simulink model "General_posicion1"  (R2020b)
settings: Solver=ode5  StartTime=0.0  StopTime=inf  RelTol=1e-3
undefined symbols (not defined in the file): National_Instruments, PCI
libraries: simulink x4, pid_lib x3, fuzblock x2, sldrtlib x2
settings Model: SimulationMode=external  Creator=Usuario_UMA  LastModifiedBy=alumnoic06
settings RTWCC: Description=Simulink Desktop Real-Time  SystemTargetFile=sldrt.tlc  TemplateMakefile=sldrt.tmf  RTWCompilerOptimization=on
settings CodeAppCC: MaxIdLength=95
settings SimulinkDesktopRealTimeCC: TargetPreCompLibLocation=C:\Program Files\MATLAB\R2020\toolbox\sldrt\lib\win64

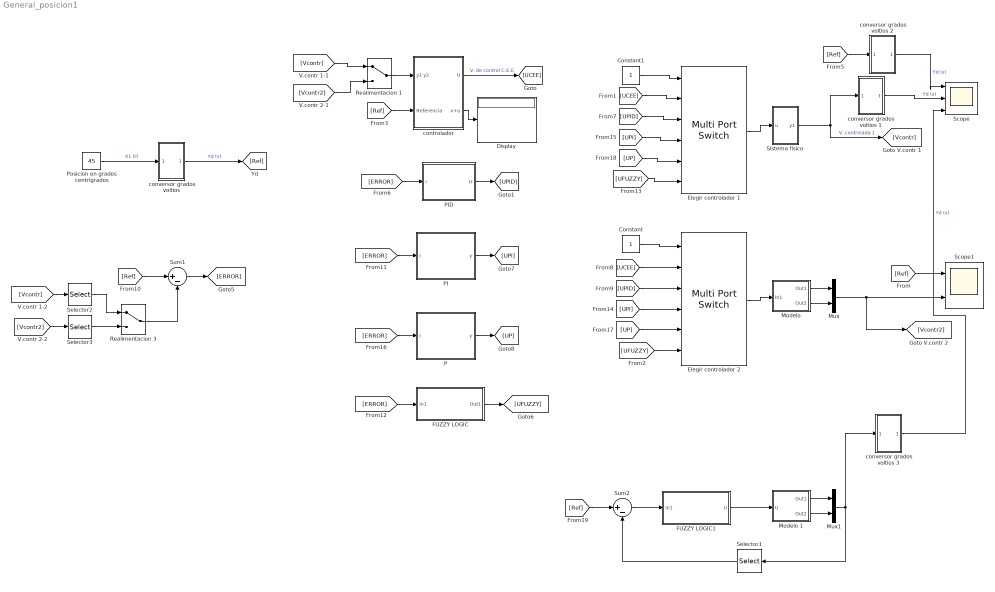
== system General_posicion1 ==
  Constant : Constant
  Constant1 : Constant
  Display : Display
  Elegir controlador 1 : MultiPortSwitch  Inputs=5
  Elegir controlador 2 : MultiPortSwitch  Inputs=5
  FUZZY LOGIC : Subsystem
  FUZZY LOGIC1 : Subsystem
  "Modelo " : Subsystem
  Modelo 1 : Subsystem
  Mux : Mux  Inputs=2
  Mux1 : Mux  Inputs=2
  P : Subsystem
  PI : Subsystem
  PID : Subsystem
  Posicion en grados centrigrados : Constant  Value=45
  Realimentacion 1 : ManualSwitch
  Realimentacion 3 : ManualSwitch
  Scope : Scope  NumInputPorts=3
  Scope1 : Scope  NumInputPorts=2
  Selector1 : Selector  InputPortWidth=2  IndexOptions=Index vector (dialog)  Indices=[1]  OutputSizes=1
  Selector2 : Selector  InputPortWidth=2  IndexOptions=Index vector (dialog)  Indices=[1]  OutputSizes=1
  Selector3 : Selector  InputPortWidth=2  IndexOptions=Index vector (dialog)  Indices=[1]  OutputSizes=1
  Sistema fisico : Subsystem
  Sum1 : Sum  Inputs=|+-
  Sum2 : Sum  Inputs=|+-
  controlador : Subsystem
  "conversor grados voltios " : Subsystem  mask{a=4.91, b=0}
  conversor grados voltios 1 : Subsystem  mask{a=4.91, b=0}
  conversor grados voltios 2 : Subsystem  mask{a=4.91, b=0}
  conversor grados voltios 3 : Subsystem  mask{a=4.91, b=0}
  wires:
  Posicion en grados centrigrados/1 -> "conversor grados voltios "/1(In1)  "X1 (º)"
  controlador/2(x+u) -> Display/1
  Sistema fisico/1(y1) -> conversor grados voltios 1/1(In1), [Vcontr]  "V. controlada 1"
  "conversor grados voltios "/1(Out1) -> [Ref]  "Yd (v)"
  controlador/1(U) -> [UCEE]  "V. de control C:E:E"
  "Modelo "/1(Out1) -> Mux/1
  "Modelo "/2(Out2) -> Mux/2
  Mux/1 -> [Vcontr2], Scope1/2
  Realimentacion 1/1 -> controlador/1(y1 y2)
  [Ref] -> Scope1/1
  [Vcontr] -> Realimentacion 1/1
  [Vcontr2] -> Realimentacion 1/2
  [Ref] -> controlador/2(Referencia)
  Elegir controlador 2/1 -> "Modelo "/1(In1)
  Elegir controlador 1/1 -> Sistema fisico/1(u)
  PID/1(U) -> [UPID]
  [UCEE] -> Elegir controlador 1/2
  [UPID] -> Elegir controlador 1/3
  [UCEE] -> Elegir controlador 2/2
  [UPID] -> Elegir controlador 2/3
  Constant/1 -> Elegir controlador 2/1
  Constant1/1 -> Elegir controlador 1/1
  [Vcontr2] -> Selector3/1
  Selector3/1 -> Realimentacion 3/2
  [Ref] -> Sum1/1
  Realimentacion 3/1 -> Sum1/2
  Selector2/1 -> Realimentacion 3/1
  Sum1/1 -> [ERROR]
  [Vcontr] -> Selector2/1
  [ERROR] -> PID/1(r)
  [ERROR] -> FUZZY LOGIC/1(In1)
  FUZZY LOGIC/1(Out1) -> [UFUZZY]
  [UFUZZY] -> Elegir controlador 2/6
  [UFUZZY] -> Elegir controlador 1/6
  [ERROR] -> PI/1(r)
  PI/1(y) -> [UPI]
  [UPI] -> Elegir controlador 2/4
  [UPI] -> Elegir controlador 1/4
  [ERROR] -> P/1(r)
  P/1(y) -> [UP]
  [UP] -> Elegir controlador 2/5
  [UP] -> Elegir controlador 1/5
  conversor grados voltios 1/1(Out1) -> Scope/2  "Yd (v)"
  [Ref] -> conversor grados voltios 2/1(In1)
  conversor grados voltios 2/1(Out1) -> Scope/1  "Yd (v)"
  [Ref] -> Sum2/1
  Modelo 1/2(Out2) -> Mux1/2
  Modelo 1/1(Out1) -> Mux1/1
  Selector1/1 -> Sum2/2
  Mux1/1 -> Selector1/1, conversor grados voltios 3/1(In1)
  conversor grados voltios 3/1(Out1) -> Scope/3  "Yd (v)"
  Sum2/1 -> FUZZY LOGIC1/1(In1)
  FUZZY LOGIC1/1(U) -> Modelo 1/1(U)

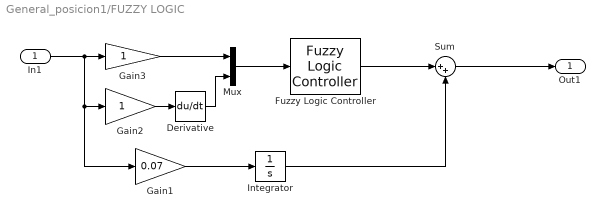
== system General_posicion1/FUZZY LOGIC ==
  In1 : Inport
  Derivative : Derivative
  Fuzzy Logic Controller : fuzblock/Fuzzy Logic  Controller  FIS='FUZZY1b.fis'  OutputSampleNumber=101  DataType=double  FuzzifiedInputs=off  RuleFiringStrengths=off  RuleOutputs=off  AggregatedOutputs=off  SimulateUsing=Interpreted execution  OutOfRangeInputValueMessage=warning  NoRuleFiredMessage=warning  EmptyOutputFuzzySetMessage=warning
  Gain1 : Gain  Gain=0.07
  Gain2 : Gain
  Gain3 : Gain
  Integrator : Integrator
  Mux : Mux  Inputs=2
  Sum : Sum  Inputs=|++
  Out1 : Outport
  wires:
  Derivative/1 -> Mux/2
  In1/1 -> Gain3/1, Gain1/1, Gain2/1
  Mux/1 -> Fuzzy Logic Controller/1
  Gain3/1 -> Mux/1
  Gain2/1 -> Derivative/1
  Gain1/1 -> Integrator/1
  Fuzzy Logic Controller/1 -> Sum/1
  Sum/1 -> Out1/1
  Integrator/1 -> Sum/2

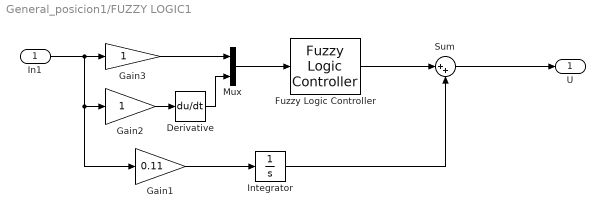
== system General_posicion1/FUZZY LOGIC1 ==
  In1 : Inport
  Derivative : Derivative
  Fuzzy Logic Controller : fuzblock/Fuzzy Logic  Controller  FIS='FUZZY1b.fis'  OutputSampleNumber=101  DataType=double  FuzzifiedInputs=off  RuleFiringStrengths=off  RuleOutputs=off  AggregatedOutputs=off  SimulateUsing=Interpreted execution  OutOfRangeInputValueMessage=warning  NoRuleFiredMessage=warning  EmptyOutputFuzzySetMessage=warning
  Gain1 : Gain  Gain=0.11
  Gain2 : Gain
  Gain3 : Gain
  Integrator : Integrator
  Mux : Mux  Inputs=2
  Sum : Sum  Inputs=|++
  U : Outport
  wires:
  Derivative/1 -> Mux/2
  In1/1 -> Gain3/1, Gain1/1, Gain2/1
  Mux/1 -> Fuzzy Logic Controller/1
  Gain3/1 -> Mux/1
  Gain2/1 -> Derivative/1
  Gain1/1 -> Integrator/1
  Fuzzy Logic Controller/1 -> Sum/1
  Sum/1 -> U/1
  Integrator/1 -> Sum/2

== system General_posicion1/Modelo  ==
  In1 : Inport
  Transfer Fcn : TransferFcn  Numerator=[114.486]  Denominator=[1 7.35 0]
  Transfer Fcn1 : TransferFcn  Numerator=[19.12]  Denominator=[1 7.35]
  Out1 : Outport
  Out2 : Outport  Port=2
  wires:
  In1/1 -> Transfer Fcn1/1, Transfer Fcn/1
  Transfer Fcn/1 -> Out1/1
  Transfer Fcn1/1 -> Out2/1

== system General_posicion1/Modelo 1 ==
  U : Inport
  Transfer Fcn : TransferFcn  Numerator=[114.486]  Denominator=[1 7.35 0]
  Transfer Fcn1 : TransferFcn  Numerator=[19.12]  Denominator=[1 7.35]
  Out1 : Outport
  Out2 : Outport  Port=2
  wires:
  U/1 -> Transfer Fcn1/1, Transfer Fcn/1
  Transfer Fcn/1 -> Out1/1
  Transfer Fcn1/1 -> Out2/1

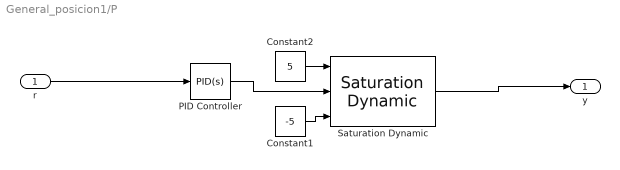
== system General_posicion1/P ==
  r : Inport
  Constant1 : Constant  Value=-5
  Constant2 : Constant  Value=5
  PID Controller : pid_lib/PID Controller  Controller=PID  Form=Parallel  TimeDomain=Continuous-time  UseExternalTs=off  SampleTime=-1  IntegratorMethod=Forward Euler  FilterMethod=Forward Euler  ControllerParametersSource=internal  P=0.5  I=0.2  D=0  UseFilter=on  N=100  TunerSelectOption=Transfer Function Based (PID Tuner App)  InitialConditionSource=internal  InitialConditionForIntegrator=0  InitialConditionForFilter=0  DifferentiatorICPrevScaledInput=0  ExternalReset=none  TrackingMode=off  Kt=1  LimitOutput=off  SatLimitsSource=internal  UpperSaturationLimit=inf  LowerSaturationLimit=-inf  LinearizeAsGain=on  AntiWindupMode=none  Kb=1  POutMin=[]  POutMax=[]  IOutMin=[]  IOutMax=[]  DOutMin=[]  DOutMax=[]  NOutMin=[]  NOutMax=[]  SumOutMin=[]  SumOutMax=[]  SaturationOutMin=[]  SaturationOutMax=[]  PParamMin=[]  PParamMax=[]  IParamMin=[]  IParamMax=[]  DParamMin=[]  DParamMax=[]  NParamMin=[]  NParamMax=[]  KbParamMin=[]  KbParamMax=[]  KtParamMin=[]  KtParamMax=[]  KbOutMin=[]  KbOutMax=[]  KtOutMin=[]  KtOutMax=[]  IntegratorOutMin=[]  IntegratorOutMax=[]  FilterOutMin=[]  FilterOutMax=[]  SumI1OutMin=[]  SumI1OutMax=[]  SumI2OutMin=[]  SumI2OutMax=[]  SumI3OutMin=[]  SumI3OutMax=[]  SumI4OutMin=[]  SumI4OutMax=[]  SumDOutMin=[]  SumDOutMax=[]  DifferentiatorOutMin=[]  DifferentiatorOutMax=[]  FilterDiffOutCoefMin=[]  FilterDiffOutCoefMax=[]  ReciprocalOutMin=[]  ReciprocalOutMax=[]  SumDenOutMin=[]  SumDenOutMax=[]  SumNumOutMin=[]  SumNumOutMax=[]  DivideOutMin=[]  DivideOutMax=[]  UdiffTsProdOutMin=[]  UdiffTsProdOutMax=[]  NTsProdOutMin=[]  NTsProdOutMax=[]  UintegralTsProdOutMin=[]  UintegralTsProdOutMax=[]  UngainTsProdOutMin=[]  UngainTsProdOutMax=[]  IntegratorContinuousStateAttributes=''  IntegratorStateMustResolveToSignalObject=off  IntegratorRTWStateStorageClass=Auto  FilterContinuousStateAttributes=''  FilterStateMustResolveToSignalObject=off  FilterRTWStateStorageClass=Auto  ParallelPVariant=InternalParameters  IdealPVariant=Disabled  IVariant=InternalParameters  DVariant=InternalParameters  IntegratorVariant=Continuous  SatVariant=Disabled  AWVariant=Passthrough  PCopyVariant=Disabled  TRVariant=Disabled  FdbkBlocksVariant=Forward  IdealPFdbkVariant=Disabled  SatFdbkVariant=Disabled  DerivativeFilterVariant=ContFilter  NVariant=InternalParameters  NCopyVariant=Disabled  FilterICVariant=InternalICsFilter  IntegratorICVariant=InternalICs  ExternalResetVariant=Disabled  TRSumVariant=Passthrough  SumFdbkVariant=Disabled  SumVariant=Sum_PID  TsampFilterVariant=InternalTs  TsampNgainVariant=Passthrough  TsampIntegralVariant=Passthrough  ExternalSaturationOutDataTypeStr=Inherit: Same as second input
  Saturation Dynamic : simulink/Discontinuities/Saturation Dynamic  OutMin=-5  OutMax=5  OutDataTypeStr=Inherit: Same as second input  OutDataType=fixdt(1, 16)  OutScaling=2^-10  DoSatur=off
      settings: LockScale=on
  y : Outport
  wires:
  r/1 -> PID Controller/1
  PID Controller/1 -> Saturation Dynamic/2
  Constant2/1 -> Saturation Dynamic/1
  Constant1/1 -> Saturation Dynamic/3
  Saturation Dynamic/1 -> y/1

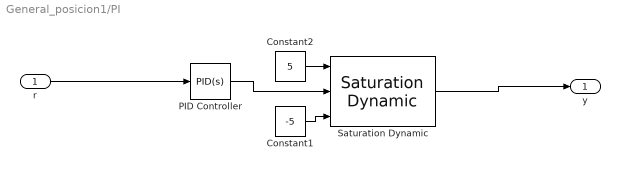
== system General_posicion1/PI ==
  r : Inport
  Constant1 : Constant  Value=-5
  Constant2 : Constant  Value=5
  PID Controller : pid_lib/PID Controller  Controller=PID  Form=Parallel  TimeDomain=Continuous-time  UseExternalTs=off  SampleTime=-1  IntegratorMethod=Forward Euler  FilterMethod=Forward Euler  ControllerParametersSource=internal  P=0.5  I=0.2  D=0  UseFilter=on  N=100  TunerSelectOption=Transfer Function Based (PID Tuner App)  InitialConditionSource=internal  InitialConditionForIntegrator=0  InitialConditionForFilter=0  DifferentiatorICPrevScaledInput=0  ExternalReset=none  TrackingMode=off  Kt=1  LimitOutput=off  SatLimitsSource=internal  UpperSaturationLimit=inf  LowerSaturationLimit=-inf  LinearizeAsGain=on  AntiWindupMode=none  Kb=1  POutMin=[]  POutMax=[]  IOutMin=[]  IOutMax=[]  DOutMin=[]  DOutMax=[]  NOutMin=[]  NOutMax=[]  SumOutMin=[]  SumOutMax=[]  SaturationOutMin=[]  SaturationOutMax=[]  PParamMin=[]  PParamMax=[]  IParamMin=[]  IParamMax=[]  DParamMin=[]  DParamMax=[]  NParamMin=[]  NParamMax=[]  KbParamMin=[]  KbParamMax=[]  KtParamMin=[]  KtParamMax=[]  KbOutMin=[]  KbOutMax=[]  KtOutMin=[]  KtOutMax=[]  IntegratorOutMin=[]  IntegratorOutMax=[]  FilterOutMin=[]  FilterOutMax=[]  SumI1OutMin=[]  SumI1OutMax=[]  SumI2OutMin=[]  SumI2OutMax=[]  SumI3OutMin=[]  SumI3OutMax=[]  SumI4OutMin=[]  SumI4OutMax=[]  SumDOutMin=[]  SumDOutMax=[]  DifferentiatorOutMin=[]  DifferentiatorOutMax=[]  FilterDiffOutCoefMin=[]  FilterDiffOutCoefMax=[]  ReciprocalOutMin=[]  ReciprocalOutMax=[]  SumDenOutMin=[]  SumDenOutMax=[]  SumNumOutMin=[]  SumNumOutMax=[]  DivideOutMin=[]  DivideOutMax=[]  UdiffTsProdOutMin=[]  UdiffTsProdOutMax=[]  NTsProdOutMin=[]  NTsProdOutMax=[]  UintegralTsProdOutMin=[]  UintegralTsProdOutMax=[]  UngainTsProdOutMin=[]  UngainTsProdOutMax=[]  IntegratorContinuousStateAttributes=''  IntegratorStateMustResolveToSignalObject=off  IntegratorRTWStateStorageClass=Auto  FilterContinuousStateAttributes=''  FilterStateMustResolveToSignalObject=off  FilterRTWStateStorageClass=Auto  ParallelPVariant=InternalParameters  IdealPVariant=Disabled  IVariant=InternalParameters  DVariant=InternalParameters  IntegratorVariant=Continuous  SatVariant=Disabled  AWVariant=Passthrough  PCopyVariant=Disabled  TRVariant=Disabled  FdbkBlocksVariant=Forward  IdealPFdbkVariant=Disabled  SatFdbkVariant=Disabled  DerivativeFilterVariant=ContFilter  NVariant=InternalParameters  NCopyVariant=Disabled  FilterICVariant=InternalICsFilter  IntegratorICVariant=InternalICs  ExternalResetVariant=Disabled  TRSumVariant=Passthrough  SumFdbkVariant=Disabled  SumVariant=Sum_PID  TsampFilterVariant=InternalTs  TsampNgainVariant=Passthrough  TsampIntegralVariant=Passthrough  ExternalSaturationOutDataTypeStr=Inherit: Same as second input
  Saturation Dynamic : simulink/Discontinuities/Saturation Dynamic  OutMin=-5  OutMax=5  OutDataTypeStr=Inherit: Same as second input  OutDataType=fixdt(1, 16)  OutScaling=2^-10  DoSatur=off
      settings: LockScale=on
  y : Outport
  wires:
  r/1 -> PID Controller/1
  PID Controller/1 -> Saturation Dynamic/2
  Constant2/1 -> Saturation Dynamic/1
  Constant1/1 -> Saturation Dynamic/3
  Saturation Dynamic/1 -> y/1

== system General_posicion1/PID ==
  r : Inport
  PID Controller : pid_lib/PID Controller  Controller=PID  Form=Parallel  TimeDomain=Continuous-time  UseExternalTs=off  SampleTime=-1  IntegratorMethod=Forward Euler  FilterMethod=Forward Euler  ControllerParametersSource=internal  P=0.8  I=1  D=0.1  UseFilter=on  N=100  TunerSelectOption=Transfer Function Based (PID Tuner App)  InitialConditionSource=internal  InitialConditionForIntegrator=0  InitialConditionForFilter=0  DifferentiatorICPrevScaledInput=0  ExternalReset=none  TrackingMode=off  Kt=1  LimitOutput=on  SatLimitsSource=internal  UpperSaturationLimit=inf  LowerSaturationLimit=-inf  LinearizeAsGain=on  AntiWindupMode=clamping  Kb=1  POutMin=[]  POutMax=[]  IOutMin=[]  IOutMax=[]  DOutMin=[]  DOutMax=[]  NOutMin=[]  NOutMax=[]  SumOutMin=[]  SumOutMax=[]  SaturationOutMin=[]  SaturationOutMax=[]  PParamMin=[]  PParamMax=[]  IParamMin=[]  IParamMax=[]  DParamMin=[]  DParamMax=[]  NParamMin=[]  NParamMax=[]  KbParamMin=[]  KbParamMax=[]  KtParamMin=[]  KtParamMax=[]  KbOutMin=[]  KbOutMax=[]  KtOutMin=[]  KtOutMax=[]  IntegratorOutMin=[]  IntegratorOutMax=[]  FilterOutMin=[]  FilterOutMax=[]  SumI1OutMin=[]  SumI1OutMax=[]  SumI2OutMin=[]  SumI2OutMax=[]  SumI3OutMin=[]  SumI3OutMax=[]  SumI4OutMin=[]  SumI4OutMax=[]  SumDOutMin=[]  SumDOutMax=[]  DifferentiatorOutMin=[]  DifferentiatorOutMax=[]  FilterDiffOutCoefMin=[]  FilterDiffOutCoefMax=[]  ReciprocalOutMin=[]  ReciprocalOutMax=[]  SumDenOutMin=[]  SumDenOutMax=[]  SumNumOutMin=[]  SumNumOutMax=[]  DivideOutMin=[]  DivideOutMax=[]  UdiffTsProdOutMin=[]  UdiffTsProdOutMax=[]  NTsProdOutMin=[]  NTsProdOutMax=[]  UintegralTsProdOutMin=[]  UintegralTsProdOutMax=[]  UngainTsProdOutMin=[]  UngainTsProdOutMax=[]  IntegratorContinuousStateAttributes=''  IntegratorStateMustResolveToSignalObject=off  IntegratorRTWStateStorageClass=Auto  FilterContinuousStateAttributes=''  FilterStateMustResolveToSignalObject=off  FilterRTWStateStorageClass=Auto  ParallelPVariant=InternalParameters  IdealPVariant=Disabled  IVariant=InternalParameters  DVariant=InternalParameters  IntegratorVariant=Continuous  SatVariant=Enabled  AWVariant=ContClampingParallel  PCopyVariant=Disabled  TRVariant=Disabled  FdbkBlocksVariant=Forward  IdealPFdbkVariant=Disabled  SatFdbkVariant=Disabled  DerivativeFilterVariant=ContFilter  NVariant=InternalParameters  NCopyVariant=Disabled  FilterICVariant=InternalICsFilter  IntegratorICVariant=InternalICs  ExternalResetVariant=Disabled  TRSumVariant=Passthrough  SumFdbkVariant=Disabled  SumVariant=Sum_PID  TsampFilterVariant=InternalTs  TsampNgainVariant=Passthrough  TsampIntegralVariant=Passthrough  ExternalSaturationOutDataTypeStr=Inherit: Same as second input
  saturador : Subsystem
  U : Outport
  wires:
  PID Controller/1 -> saturador/1(u)
  r/1 -> PID Controller/1
  saturador/1(U) -> U/1

== system General_posicion1/Sistema fisico ==
  u : Inport
  Analog Input2 : sldrtlib/Analog Input  SampleTime=0.01  MaxMissedTicks=10  ShowMissedTicks=off  YieldWhenWaiting=off  DrvName=National_Instruments/PCI-6014  DrvAddress=4294967295  DrvOptions=[2 0 0 0 0 0]  Channels=[1,2]  RangeMode=1  VoltRange=1  DataType=1
      settings: AttributesFormatString=National Instruments\nPCI-6014 [auto]
  Analog Output : sldrtlib/Analog Output  SampleTime=0.01  MaxMissedTicks=10  ShowMissedTicks=off  YieldWhenWaiting=off  DrvName=National_Instruments/PCI-6014  DrvAddress=4294967295  DrvOptions=[2 0 0 0 0 0]  Channels=1  RangeMode=1  VoltRange=1  InitialValue=[]  FinalValue=[]
      settings: AttributesFormatString=National Instruments\nPCI-6014 [auto]
  y1 : Outport
  wires:
  u/1 -> Analog Output/1
  Analog Input2/1 -> y1/1  "Original signal"

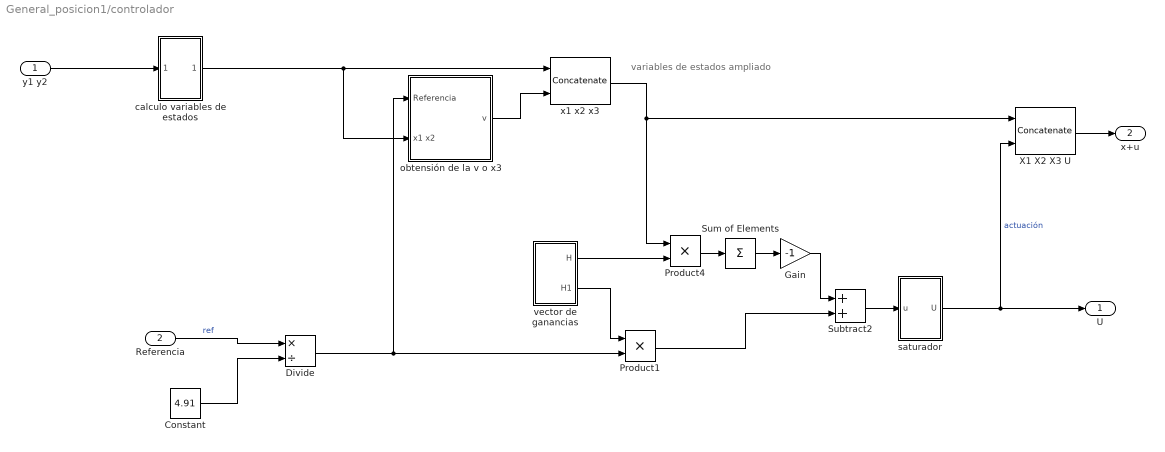
== system General_posicion1/controlador ==
  note: variables de estados ampliado
  y1 y2 : Inport  OutDataTypeStr=double
  Referencia : Inport  Port=2
  Constant : Constant  Value=4.91
  Divide : Product  Inputs=*/
  Gain : Gain  Gain=-1
  Product1 : Product
  Product4 : Product
  Subtract2 : Sum  OutDataTypeStr=double
  Sum of Elements : Sum  Inputs=+
  X1 X2 X3 U : Concatenate  ConcatenateDimension=2
  "calculo variables de estados " : Subsystem  mask{a=4.91, b=0.8179}
  obtensión de la v o x3 : Subsystem
  saturador : Subsystem
  vector de ganancias : Subsystem  mask{h1=15.349, h2=0.76, h3=-0.019}
  x1 x2 x3 : Concatenate  ConcatenateDimension=2
  U : Outport  OutDataTypeStr=double
  x+u : Outport  Port=2
  wires:
  Product4/1 -> Sum of Elements/1
  Gain/1 -> Subtract2/1
  vector de ganancias/1(H) -> Product4/2
  Subtract2/1 -> saturador/1(u)
  Sum of Elements/1 -> Gain/1
  Referencia/1 -> Divide/1  "ref"
  saturador/1(U) -> U/1, X1 X2 X3 U/2  "actuación"
  X1 X2 X3 U/1 -> x+u/1
  x1 x2 x3/1 -> X1 X2 X3 U/1, Product4/1
  y1 y2/1 -> "calculo variables de estados "/1(In1)
  "calculo variables de estados "/1("[x1 x2]") -> obtensión de la v o x3/2(x1 x2), x1 x2 x3/1
  Constant/1 -> Divide/2
  Divide/1 -> obtensión de la v o x3/1(Referencia), Product1/2
  vector de ganancias/2(H1) -> Product1/1
  Product1/1 -> Subtract2/2
  obtensión de la v o x3/1(v) -> x1 x2 x3/2

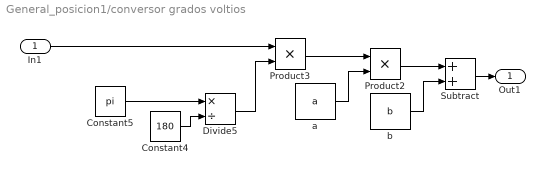
== system General_posicion1/conversor grados voltios  ==
  In1 : Inport
  Constant4 : Constant  Value=180
  Constant5 : Constant  Value=pi
  Divide5 : Product  Inputs=*/
  Product2 : Product
  Product3 : Product
  Subtract : Sum
  a : Constant  Value=a
  b : Constant  Value=b
  Out1 : Outport
  wires:
  b/1 -> Subtract/2
  Product3/1 -> Product2/1
  Constant4/1 -> Divide5/2
  In1/1 -> Product3/1
  Product2/1 -> Subtract/1
  a/1 -> Product2/2
  Constant5/1 -> Divide5/1
  Divide5/1 -> Product3/2
  Subtract/1 -> Out1/1

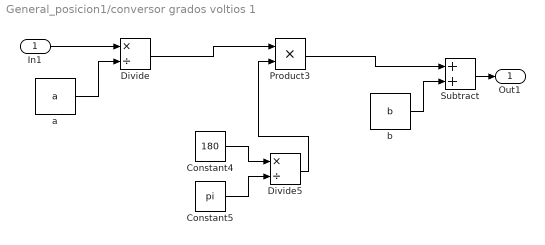
== system General_posicion1/conversor grados voltios 1 ==
  In1 : Inport
  Constant4 : Constant  Value=180
  Constant5 : Constant  Value=pi
  Divide : Product  Inputs=*/
  Divide5 : Product  Inputs=*/
  Product3 : Product
  Subtract : Sum
  a : Constant  Value=a
  b : Constant  Value=b
  Out1 : Outport
  wires:
  b/1 -> Subtract/2
  Product3/1 -> Subtract/1
  Divide5/1 -> Product3/2
  Subtract/1 -> Out1/1
  In1/1 -> Divide/1
  a/1 -> Divide/2
  Divide/1 -> Product3/1
  Constant4/1 -> Divide5/1
  Constant5/1 -> Divide5/2

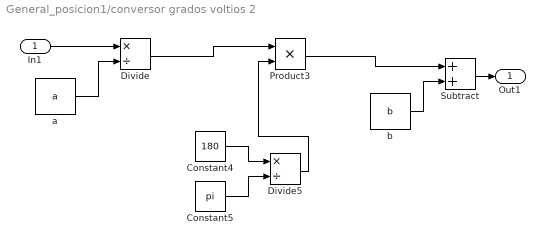
== system General_posicion1/conversor grados voltios 2 ==
  In1 : Inport
  Constant4 : Constant  Value=180
  Constant5 : Constant  Value=pi
  Divide : Product  Inputs=*/
  Divide5 : Product  Inputs=*/
  Product3 : Product
  Subtract : Sum
  a : Constant  Value=a
  b : Constant  Value=b
  Out1 : Outport
  wires:
  b/1 -> Subtract/2
  Product3/1 -> Subtract/1
  Divide5/1 -> Product3/2
  Subtract/1 -> Out1/1
  In1/1 -> Divide/1
  a/1 -> Divide/2
  Divide/1 -> Product3/1
  Constant4/1 -> Divide5/1
  Constant5/1 -> Divide5/2

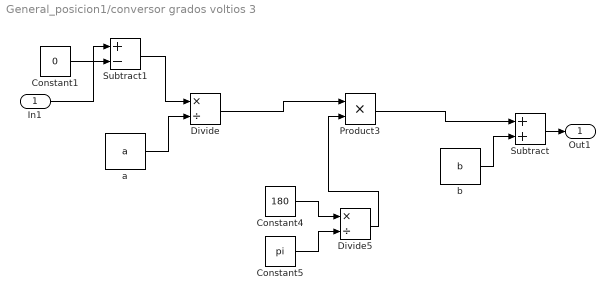
== system General_posicion1/conversor grados voltios 3 ==
  In1 : Inport
  Constant1 : Constant  Value=0
  Constant4 : Constant  Value=180
  Constant5 : Constant  Value=pi
  Divide : Product  Inputs=*/
  Divide5 : Product  Inputs=*/
  Product3 : Product
  Subtract : Sum
  Subtract1 : Sum  Inputs=+-
  a : Constant  Value=a
  b : Constant  Value=b
  Out1 : Outport
  wires:
  b/1 -> Subtract/2
  Product3/1 -> Subtract/1
  Divide5/1 -> Product3/2
  Subtract/1 -> Out1/1
  In1/1 -> Subtract1/1
  a/1 -> Divide/2
  Divide/1 -> Product3/1
  Constant4/1 -> Divide5/1
  Constant5/1 -> Divide5/2
  Constant1/1 -> Subtract1/2
  Subtract1/1 -> Divide/1

== system General_posicion1/PID/saturador ==
  u : Inport  OutDataTypeStr=double
  Constant1 : Constant  Value=-5
  Constant2 : Constant  Value=5
  Saturation Dynamic : simulink/Discontinuities/Saturation Dynamic  OutMin=-5  OutMax=5  OutDataTypeStr=Inherit: Same as second input  OutDataType=fixdt(1, 16)  OutScaling=2^-10  DoSatur=off
  U : Outport  OutDataTypeStr=double
  wires:
  u/1 -> Saturation Dynamic/2
  Constant2/1 -> Saturation Dynamic/1
  Saturation Dynamic/1 -> U/1
  Constant1/1 -> Saturation Dynamic/3

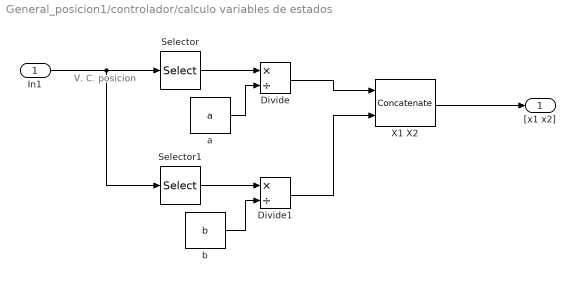
== system General_posicion1/controlador/calculo variables de estados  ==
  note: V. C. posicion
  In1 : Inport
  Divide : Product  Inputs=*/
  Divide1 : Product  Inputs=*/
  Selector : Selector  InputPortWidth=2  IndexOptions=Index vector (dialog)  Indices=[1]  OutputSizes=1
  Selector1 : Selector  InputPortWidth=2  IndexOptions=Index vector (dialog)  Indices=[2]  OutputSizes=1
  "X1 X2 " : Concatenate  ConcatenateDimension=2
  a : Constant  Value=a
  b : Constant  Value=b
  "[x1 x2]" : Outport
  wires:
  In1/1 -> Selector1/1, Selector/1
  "X1 X2 "/1 -> "[x1 x2]"/1
  Selector/1 -> Divide/1
  a/1 -> Divide/2
  Selector1/1 -> Divide1/1
  b/1 -> Divide1/2
  Divide/1 -> "X1 X2 "/1
  Divide1/1 -> "X1 X2 "/2

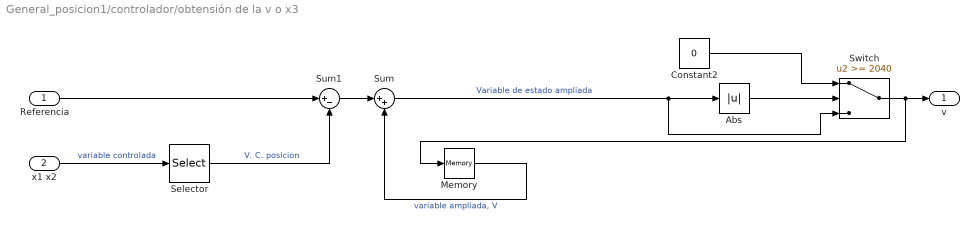
== system General_posicion1/controlador/obtensión de la v o x3 ==
  Referencia : Inport
  x1 x2 : Inport  Port=2  PortDimensions=2
  Abs : Abs
  Constant2 : Constant  Value=0
  Memory : Memory  InheritSampleTime=on  LinearizeAsDelay=on
  Selector : Selector  InputPortWidth=2  IndexOptions=Index vector (dialog)  Indices=[1]  OutputSizes=1
  Sum : Sum  Inputs=|++
  Sum1 : Sum  Inputs=|+-
  Switch : Switch  Threshold=2040
  v : Outport
  wires:
  Referencia/1 -> Sum1/1
  Sum/1 -> Switch/3, Abs/1  "Variable de estado ampliada"
  Sum1/1 -> Sum/1
  Memory/1 -> Sum/2  "variable ampliada, V"
  x1 x2/1 -> Selector/1  "variable controlada"
  Selector/1 -> Sum1/2  "V. C. posicion"
  Constant2/1 -> Switch/1
  Abs/1 -> Switch/2
  Switch/1 -> Memory/1, v/1

== system General_posicion1/controlador/saturador ==
  u : Inport  OutDataTypeStr=double
  Constant1 : Constant  Value=-5
  Constant2 : Constant  Value=5
  Saturation Dynamic : simulink/Discontinuities/Saturation Dynamic  OutMin=-5  OutMax=5  OutDataTypeStr=Inherit: Same as second input  OutDataType=fixdt(1, 16)  OutScaling=2^-10  DoSatur=off
  U : Outport  OutDataTypeStr=double
  wires:
  u/1 -> Saturation Dynamic/2
  Constant2/1 -> Saturation Dynamic/1
  Saturation Dynamic/1 -> U/1
  Constant1/1 -> Saturation Dynamic/3

== system General_posicion1/controlador/vector de ganancias ==
  Ht : Concatenate  NumInputs=3  ConcatenateDimension=2
  h1 : Constant  Value=h1
  h2 : Constant  Value=h2
  h3 : Constant  Value=h3
  H : Outport
  H1 : Outport  Port=2
  wires:
  h1/1 -> H1/1, Ht/1
  h2/1 -> Ht/2
  Ht/1 -> H/1
  h3/1 -> Ht/3
